simulink model "lookup1"  (R2021b)
settings: Solver=VariableStepAuto  StartTime=0.0  StopTime=6  RelTol=1e-3
undefined symbols (not defined in the file or in its folder): Number, Number1, SA, Values
libraries: simulink x1
settings Model: Creator=syedfazal  LastModifiedBy=GL62

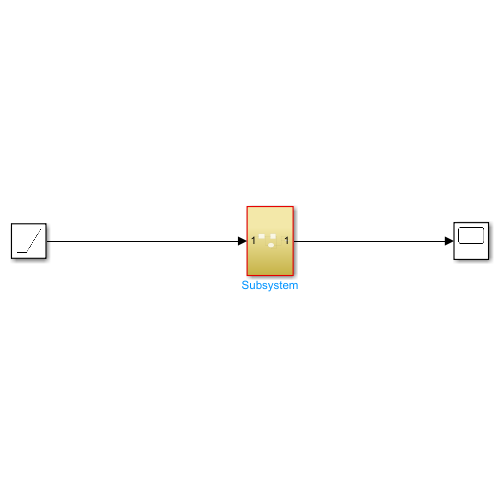
[thumbnail: Simulink's stored preview of the top-level diagram]
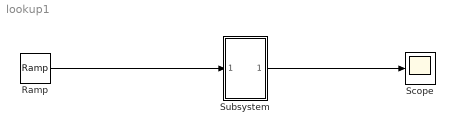
== system lookup1 ==
  Ramp : simulink/Sources/Ramp  slope=1  start=0  InitialOutput=0
  Scope : Scope
  Subsystem : Subsystem
  wires:
  Ramp/1 -> Subsystem/1(In1)
  Subsystem/1(Out1) -> Scope/1

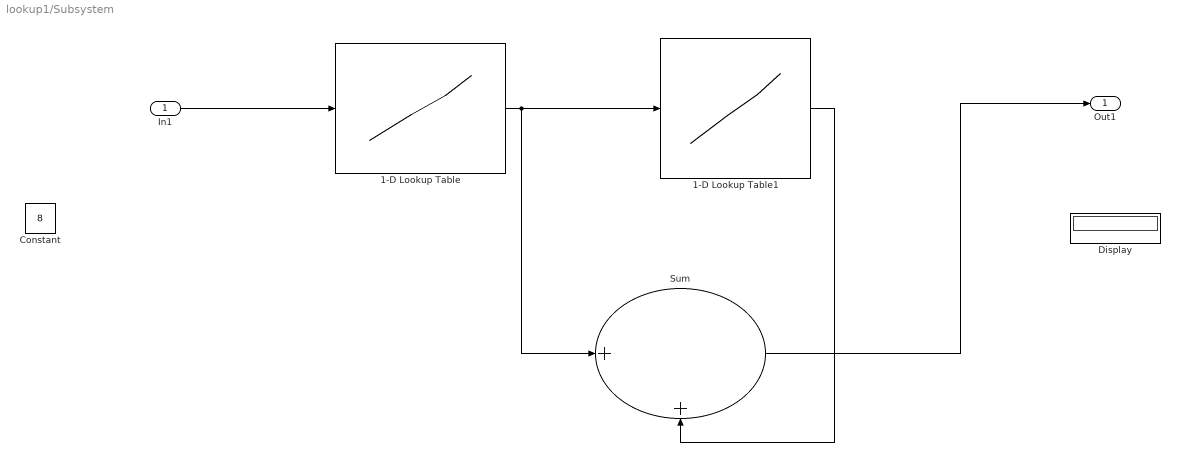
== system lookup1/Subsystem ==
  In1 : Inport
  1-D Lookup Table : Lookup_n-D  NumberOfTableDimensions=1  BreakpointsForDimension1=Number  Table=Values  InterpMethod=Cubic spline  InternalRulePriority=Speed  RndMeth=Simplest  InputSameDT=on
  1-D Lookup Table1 : Lookup_n-D  NumberOfTableDimensions=1  BreakpointsForDimension1=Number1  Table=SA  InterpMethod=Cubic spline  InternalRulePriority=Speed  RndMeth=Simplest  InputSameDT=on
  Constant : Constant  Value=8
  Display : Display
  Sum : Sum  Inputs=|++
  Out1 : Outport
  wires:
  1-D Lookup Table1/1 -> Sum/2
  Sum/1 -> Out1/1
  1-D Lookup Table/1 -> Sum/1, 1-D Lookup Table1/1
  In1/1 -> 1-D Lookup Table/1
